simulink model "ACtoDC_WPT_DC_two_phase"  (R2018a)
settings: Solver=FixedStepAuto  StartTime=0.0  StopTime=stopTime  FixedStep=sampleTime  RelTol=1e-3
InitFcn:
  | fs=150e3; %Hz
  | wo=2*pi*fs;
  | stopTime=0.1;
  | sampleTime=1e-8;
  | Lp=81e-6;
  | Lp=32e-6;
  | Ls=66e-6;
  | Cs=1/ (Ls*4*pi*pi*150e3*150e3);
  | Cp=1/ (Lp*4*pi*pi*150e3*150e3);
  | RLOAD=20
  | RLOAD=16.2
  | k=0.2;
  | M=sqrt(Lp*Ls)*k;
  | Cout=1e-6; %F
  | fs=150e3*sqrt(1+k^2); %Hz
  | Rp=0.2
libraries: powerlib x94, simulink x6, dspstat3 x1
settings Model: Creator=enes_  LastModifiedBy=enes_

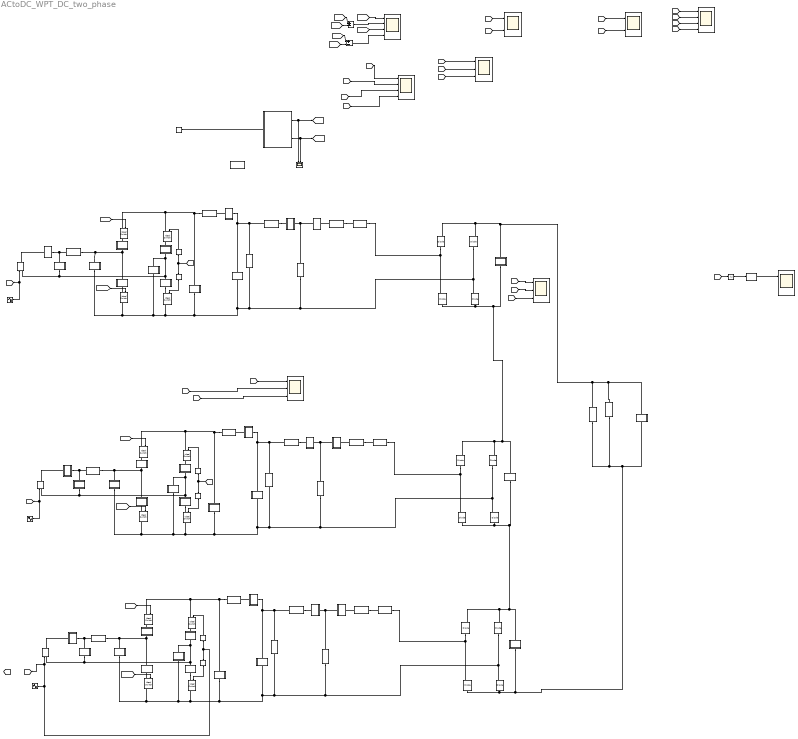
== system ACtoDC_WPT_DC_two_phase ==
  Abs : Abs
  C_TX : Subsystem
  C_TX1 : Subsystem
  C_TX10 : Subsystem
  C_TX11 : Subsystem
  C_TX12 : Subsystem
  C_TX13 : Subsystem
  C_TX14 : Subsystem
  C_TX15 : Subsystem
  C_TX16 : Subsystem
  C_TX17 : Subsystem
  C_TX18 : Subsystem
  C_TX19 : Subsystem
  C_TX2 : Subsystem
  C_TX20 : Subsystem
  C_TX21 : Subsystem
  C_TX22 : Subsystem
  C_TX23 : Subsystem
  C_TX3 : Subsystem
  C_TX4 : Subsystem
  C_TX5 : Subsystem
  C_TX6 : Subsystem
  C_TX7 : Subsystem
  C_TX8 : Subsystem
  C_TX9 : Subsystem
  Compare To Zero : simulink/Logic and Bit Operations/Compare To Zero  relop=<=  OutDataTypeStr=boolean
  Compare To Zero1 : simulink/Logic and Bit Operations/Compare To Zero  relop=>=  OutDataTypeStr=boolean
  Compare To Zero2 : simulink/Logic and Bit Operations/Compare To Zero  relop=<=  OutDataTypeStr=boolean
  Compare To Zero3 : simulink/Logic and Bit Operations/Compare To Zero  relop=>=  OutDataTypeStr=boolean
  Compare To Zero4 : simulink/Logic and Bit Operations/Compare To Zero  relop=<=  OutDataTypeStr=boolean
  Compare To Zero5 : simulink/Logic and Bit Operations/Compare To Zero  relop=>=  OutDataTypeStr=boolean
  Constant2 : Constant  Value=fs
  Controlled Voltage Source : powerlib/Electrical Sources/Controlled Voltage Source  Initialize=on  Source_Type=AC  Amplitude=0  Phase=0  Frequency=0  Measurements=None
  Controlled Voltage Source1 : powerlib/Electrical Sources/Controlled Voltage Source  Initialize=on  Source_Type=AC  Amplitude=0  Phase=0  Frequency=0  Measurements=None
  Controlled Voltage Source2 : powerlib/Electrical Sources/Controlled Voltage Source  Initialize=on  Source_Type=AC  Amplitude=0  Phase=0  Frequency=0  Measurements=None
  Diode{,1..11} (12 alike) : powerlib/Power Electronics/Diode  Ron=0.001  Lon=0  Vf=0.8  IC=0  UseSnubber=0  Rs=500  Cs=250e-9  Measurements=on
  Ideal Switch{,1..11} (12 alike) : powerlib/Power Electronics/Ideal Switch  Ron=0.01  Lon=0  IC=0  Rs=1e5  Cs=inf  Measurements=on
  Mean : dspstat3/Mean  run=on  InputProcessing=Columns as channels (frame based)  reset_popup=None  directionMode=Each column  dimension=1  roiEnable=off  roiType=Rectangles  roiPortion=Entire ROI  roiOutput=Individual statistics for each ROI  roiFlag=off  roundingMode=Floor  overflowMode=off  outputDataTypeStr=Inherit: Same as accumulator  outputMin=[]  outputMax=[]  outputLastDataTypeStr=Inherit: Same as accumulator
  Minus : Sum  Inputs=+-
  Minus1 : Sum  Inputs=+-
  Scope1 : Scope  NumInputPorts=2
  Series RLC Branch1 : powerlib/Elements/Series RLC Branch  LConnTagsString=__new0  RConnTagsString=__new0  BranchType=R  Resistance=RLOAD/2  Inductance=Lp  SetiL0=off  InitialCurrent=0  Capacitance=Cp  Setx0=off  InitialVoltage=0  Measurements=None
  Series RLC Branch10 : powerlib/Elements/Series RLC Branch  LConnTagsString=__new0  RConnTagsString=__new0  BranchType=R  Resistance=0.01  Inductance=Lp  SetiL0=off  InitialCurrent=0  Capacitance=0.01  Setx0=off  InitialVoltage=0  Measurements=None
  Series RLC Branch11 : powerlib/Elements/Series RLC Branch  LConnTagsString=__new0  RConnTagsString=__new0  BranchType=L  Resistance=Rp  Inductance=Lp-M  SetiL0=off  InitialCurrent=0  Capacitance=Cp  Setx0=off  InitialVoltage=0  Measurements=None
  Series RLC Branch12 : powerlib/Elements/Series RLC Branch  LConnTagsString=__new0  RConnTagsString=__new0  BranchType=L  Resistance=Rp  Inductance=M  SetiL0=off  InitialCurrent=0  Capacitance=Cp  Setx0=off  InitialVoltage=0  Measurements=None
  Series RLC Branch13 : powerlib/Elements/Series RLC Branch  LConnTagsString=__new0  RConnTagsString=__new0  BranchType=R  Resistance=0.01  Inductance=Lp  SetiL0=off  InitialCurrent=0  Capacitance=0.01  Setx0=off  InitialVoltage=0  Measurements=None
  Series RLC Branch14 : powerlib/Elements/Series RLC Branch  LConnTagsString=__new0  RConnTagsString=__new0  BranchType=C  Resistance=Rp  Inductance=Lp  SetiL0=off  InitialCurrent=0  Capacitance=Cp  Setx0=off  InitialVoltage=0  Measurements=None
  Series RLC Branch15 : powerlib/Elements/Series RLC Branch  LConnTagsString=__new0  RConnTagsString=__new0  BranchType=L  Resistance=Rp  Inductance=Ls-M  SetiL0=off  InitialCurrent=0  Capacitance=Cp  Setx0=off  InitialVoltage=0  Measurements=None
  Series RLC Branch16 : powerlib/Elements/Series RLC Branch  LConnTagsString=__new0  RConnTagsString=__new0  BranchType=C  Resistance=Rp  Inductance=Lp  SetiL0=off  InitialCurrent=0  Capacitance=Cs  Setx0=off  InitialVoltage=0  Measurements=None
  Series RLC Branch17 : powerlib/Elements/Series RLC Branch  LConnTagsString=__new0  RConnTagsString=__new0  BranchType=RL  Resistance=Rp  Inductance=1500e-6  SetiL0=off  InitialCurrent=0  Capacitance=Cp  Setx0=off  InitialVoltage=0  Measurements=None
  Series RLC Branch18 : powerlib/Elements/Series RLC Branch  LConnTagsString=__new0  RConnTagsString=__new0  BranchType=R  Resistance=0.01  Inductance=Lp  SetiL0=off  InitialCurrent=0  Capacitance=0.01  Setx0=off  InitialVoltage=0  Measurements=None
  Series RLC Branch19 : powerlib/Elements/Series RLC Branch  LConnTagsString=__new0  RConnTagsString=__new0  BranchType=L  Resistance=Rp  Inductance=Lp-M  SetiL0=off  InitialCurrent=0  Capacitance=Cp  Setx0=off  InitialVoltage=0  Measurements=None
  Series RLC Branch2 : powerlib/Elements/Series RLC Branch  LConnTagsString=__new0  RConnTagsString=__new0  BranchType=L  Resistance=Rp  Inductance=Lp-M  SetiL0=off  InitialCurrent=0  Capacitance=Cp  Setx0=off  InitialVoltage=0  Measurements=None
  Series RLC Branch20 : powerlib/Elements/Series RLC Branch  LConnTagsString=__new0  RConnTagsString=__new0  BranchType=L  Resistance=Rp  Inductance=M  SetiL0=off  InitialCurrent=0  Capacitance=Cp  Setx0=off  InitialVoltage=0  Measurements=None
  Series RLC Branch21 : powerlib/Elements/Series RLC Branch  LConnTagsString=__new0  RConnTagsString=__new0  BranchType=C  Resistance=Rp  Inductance=Lp  SetiL0=off  InitialCurrent=0  Capacitance=Cp  Setx0=off  InitialVoltage=0  Measurements=None
  Series RLC Branch22 : powerlib/Elements/Series RLC Branch  LConnTagsString=__new0  RConnTagsString=__new0  BranchType=L  Resistance=Rp  Inductance=Ls-M  SetiL0=off  InitialCurrent=0  Capacitance=Cp  Setx0=off  InitialVoltage=0  Measurements=None
  Series RLC Branch23 : powerlib/Elements/Series RLC Branch  LConnTagsString=__new0  RConnTagsString=__new0  BranchType=C  Resistance=Rp  Inductance=Lp  SetiL0=off  InitialCurrent=0  Capacitance=Cs  Setx0=off  InitialVoltage=0  Measurements=None
  Series RLC Branch24 : powerlib/Elements/Series RLC Branch  LConnTagsString=__new0  RConnTagsString=__new0  BranchType=RL  Resistance=Rp  Inductance=1500e-6  SetiL0=off  InitialCurrent=0  Capacitance=Cp  Setx0=off  InitialVoltage=0  Measurements=None
  Series RLC Branch3 : powerlib/Elements/Series RLC Branch  LConnTagsString=__new0  RConnTagsString=__new0  BranchType=L  Resistance=Rp  Inductance=M  SetiL0=off  InitialCurrent=0  Capacitance=Cp  Setx0=off  InitialVoltage=0  Measurements=None
  Series RLC Branch4 : powerlib/Elements/Series RLC Branch  LConnTagsString=__new0  RConnTagsString=__new0  BranchType=C  Resistance=Rp  Inductance=Lp  SetiL0=off  InitialCurrent=0  Capacitance=Cp  Setx0=off  InitialVoltage=0  Measurements=None
  Series RLC Branch5 : powerlib/Elements/Series RLC Branch  LConnTagsString=__new0  RConnTagsString=__new0  BranchType=L  Resistance=Rp  Inductance=Ls-M  SetiL0=off  InitialCurrent=0  Capacitance=Cp  Setx0=off  InitialVoltage=0  Measurements=None
  Series RLC Branch6 : powerlib/Elements/Series RLC Branch  LConnTagsString=__new0  RConnTagsString=__new0  BranchType=C  Resistance=Rp  Inductance=Lp  SetiL0=off  InitialCurrent=0  Capacitance=Cs  Setx0=off  InitialVoltage=0  Measurements=None
  Series RLC Branch7 : powerlib/Elements/Series RLC Branch  LConnTagsString=__new0  RConnTagsString=__new0  BranchType=RL  Resistance=Rp  Inductance=1500e-6  SetiL0=off  InitialCurrent=0  Capacitance=Cp  Setx0=off  InitialVoltage=0  Measurements=None
  Series RLC Branch8 : powerlib/Elements/Series RLC Branch  LConnTagsString=__new0  RConnTagsString=__new0  BranchType=C  Resistance=RLOAD  Inductance=Lp  SetiL0=off  InitialCurrent=0  Capacitance=10e-6  Setx0=off  InitialVoltage=0  Measurements=None
  Sine Wave : Sin  Amplitude=50  Frequency=2*pi*50  SampleTime=0
  Sine Wave1 : Sin  Amplitude=50  Frequency=2*pi*50  Phase=2*pi/3  SampleTime=0
  Sine Wave2 : Sin  Amplitude=50  Frequency=2*pi*50  Phase=-2*pi/3  SampleTime=0
  Subsystem1 : Subsystem
  V-I Measurement1 : Scope  NumInputPorts=3
  V-I Measurement2 : Scope  NumInputPorts=2
  V-I Measurement3 : Scope  NumInputPorts=3
  V-I Measurement4 : Scope  NumInputPorts=3
  V-I Measurement5 : Scope  NumInputPorts=2
  V-I Measurement6 : Scope  NumInputPorts=4
  V-I Measurement7 : Scope  NumInputPorts=4
  V-I Measurement8 : Scope  NumInputPorts=2
  V-I Measurement9 : Scope  NumInputPorts=4
  V_HB : Subsystem
  V_HB1 : Subsystem
  V_HB10 : Subsystem
  V_HB11 : Subsystem
  V_HB12 : Subsystem
  V_HB13 : Subsystem
  V_HB14 : Subsystem
  V_HB15 : Subsystem
  V_HB16 : Subsystem
  V_HB17 : Subsystem
  V_HB18 : Subsystem
  V_HB2 : Subsystem
  V_HB3 : Subsystem
  V_HB4 : Subsystem
  V_HB5 : Subsystem
  V_HB6 : Subsystem
  V_HB7 : Subsystem
  V_HB8 : Subsystem
  V_HB9 : Subsystem
  powergui : powerlib/powergui  Priority=1  SimulationMode=Discrete  SampleTime=sampleTime  frequency=60  Iterations=50  frequencyindice=0  Pbase=100e6  ErrMax=1e-4  UnitsV=kV  UnitsW=MW  buscounter=0  FunctionMessages=off  echomessages=off  EnableUseOfTLC=off  CurrentSourceSwitches=off  DisableSnubberDevices=off  DisableRonSwitches=off  DisableVfSwitches=off  DisplayEquations=off  SolverType=Tustin/Backward Euler (TBE)  Interpol=off  ExternalGateDelay=off  methode=off  Ts=100  x0status=blocks  SPID=off  SwTol=0  HookPort=off  RestoreLinks=warning  ResistiveCurrentMeasurement=off  Frange=[0:2:500]  Ylog=off  Xlog=on  ShowGrid=off  save=off  variable=ZData  structure=ScopeData10  ZoomFFT=off  StartTime=0.0  cycles=2  DisplayStyle=2  fundamental=50  FreqAxis=off  MaxFrequency=100e3  frequencyindicesteady=1  RmsSteady=1  display=off
  tag scope: PWMA_TOP=global
  wires:
  [V_in] -> V-I Measurement5/2  "Vin"
  Subsystem1/2(PWMA_BOT) -> Scope1/2, [PWMA_BOT]  "TA-"
  Subsystem1/1(PWMA_TOP) -> [PWMA_TOP], Scope1/1  "TA+"
  [V_aminus] -> V-I Measurement6/1  "Va-"
  [V_aposmin] -> Minus/1
  [V_aminus] -> Minus/2
  Minus/1 -> V-I Measurement6/2  "Va+"
  [V_bminus] -> V-I Measurement6/3  "Vb-"
  [V_aposmin] -> Minus1/1
  [V_bminus] -> Minus1/2
  Minus1/1 -> V-I Measurement6/4  "Vb+"
  [I_apos] -> V-I Measurement7/1  "Ia+"
  [I_bpos] -> V-I Measurement7/2  "Ib+"
  [I_in] -> V-I Measurement5/1  "Iin"
  [V_HB] -> V-I Measurement8/1  "VHB"
  [I_HB] -> V-I Measurement8/2  "IHB"
  [V_HB] -> V-I Measurement9/1  "Vtx"
  [I_Tx] -> V-I Measurement9/2  "Itx"
  [I_Rx] -> V-I Measurement9/3  "Irx"
  [Vout] -> V-I Measurement9/4  "Vrx"
  [V_in] -> V-I Measurement1/1  "Vin"
  [Vout] -> V-I Measurement1/3  "Vout"
  [I_in] -> V-I Measurement1/2  "Iin"
  [I_bmin] -> V-I Measurement7/3  "Ib-"
  [I_amin] -> V-I Measurement7/4  "Ia-"
  Constant2/1 -> Subsystem1/1(Frequency)
  Sine Wave/1 -> [Vin], Controlled Voltage Source/1
  Compare To Zero1/1 -> Ideal Switch2/1
  Mean/1 -> V-I Measurement2/1
  [Vin] -> Compare To Zero1/1, Compare To Zero/1
  [Vout] -> Abs/1
  Abs/1 -> Mean/1
  [PWMA_BOT] -> Ideal Switch/1
  [PWMA_TOP] -> Ideal Switch1/1
  Compare To Zero/1 -> Ideal Switch3/1
  [Vin2] -> Compare To Zero3/1, Compare To Zero2/1
  Compare To Zero2/1 -> Ideal Switch7/1
  [PWMA_BOT] -> Ideal Switch4/1
  [PWMA_TOP] -> Ideal Switch5/1
  Sine Wave1/1 -> [Vin2], Controlled Voltage Source1/1
  Compare To Zero3/1 -> Ideal Switch6/1
  [Vout1] -> V-I Measurement3/1
  [Vout2] -> V-I Measurement3/2
  [Vout] -> V-I Measurement3/3
  Compare To Zero5/1 -> Ideal Switch10/1
  [PWMA_TOP] -> Ideal Switch9/1
  Sine Wave2/1 -> [Vin3], Controlled Voltage Source2/1, Compare To Zero5/1, Compare To Zero4/1
  [PWMA_BOT] -> Ideal Switch8/1
  Compare To Zero4/1 -> Ideal Switch11/1
  [I_in] -> V-I Measurement4/1  "Iin"
  [I_in2] -> V-I Measurement4/2
  [I_in3] -> V-I Measurement4/3
  connections:
  Ideal Switch/RConn1 -- Diode3/RConn1 -- Diode2/LConn1 -- Series RLC Branch3/RConn1 -- Series RLC Branch4/RConn1 -- V_HB/LConn1 -- V_HB2/LConn1 -- Ideal Switch2/RConn1 -- V_HB3/LConn1 -- V_HB7/LConn1
  Series RLC Branch4/LConn1 -- V_HB/RConn1 -- C_TX4/RConn1 -- Series RLC Branch2/LConn1
  V_HB6/RConn1 -- C_TX6/RConn1 -- Series RLC Branch7/LConn1
  Series RLC Branch13/RConn1 -- Ideal Switch1/LConn1 -- Ideal Switch3/LConn1 -- V_HB2/RConn1
  C_TX/RConn1 -- Series RLC Branch3/LConn1 -- C_TX1/LConn1
  V_HB7/RConn1 -- Series RLC Branch7/RConn1 -- C_TX5/LConn1 -- C_TX2/LConn1
  Diode/LConn1 -- Series RLC Branch6/LConn1 -- Diode1/RConn1
  Series RLC Branch5/LConn1 -- C_TX1/RConn1
  Series RLC Branch2/RConn1 -- C_TX/LConn1
  C_TX2/RConn1 -- Ideal Switch1/RConn1
  C_TX4/LConn1 -- Series RLC Branch13/LConn1
  C_TX3/RConn1 -- Ideal Switch3/RConn1
  C_TX7/RConn1 -- Ideal Switch2/LConn1
  Series RLC Branch5/RConn1 -- Series RLC Branch6/RConn1
  Ideal Switch/LConn1 -- C_TX5/RConn1
  Controlled Voltage Source/RConn1 -- C_TX6/LConn1
  Ideal Switch4/RConn1 -- V_HB11/LConn1 -- V_HB9/LConn1 -- Ideal Switch6/RConn1 -- V_HB8/LConn1 -- V_HB4/LConn1 -- Series RLC Branch14/RConn1 -- Series RLC Branch12/RConn1 -- Diode7/RConn1 -- Diode6/LConn1
  Diode4/LConn1 -- Series RLC Branch16/LConn1 -- Diode5/RConn1
  Series RLC Branch10/RConn1 -- Ideal Switch5/LConn1 -- Ideal Switch7/LConn1 -- V_HB8/RConn1
  C_TX8/RConn1 -- Series RLC Branch12/LConn1 -- C_TX9/LConn1
  V_HB11/RConn1 -- Series RLC Branch17/RConn1 -- C_TX13/LConn1 -- C_TX10/LConn1
  Diode8/RConn1 -- V_HB16/RConn1 -- V_HB5/LConn1 -- Diode5/LConn1 -- Diode7/LConn1 -- Diode10/RConn1
  Series RLC Branch14/LConn1 -- Series RLC Branch11/LConn1 -- V_HB4/RConn1 -- C_TX12/RConn1
  V_HB10/RConn1 -- C_TX14/RConn1 -- Series RLC Branch17/LConn1
  Series RLC Branch15/RConn1 -- Series RLC Branch16/RConn1
  Series RLC Branch11/RConn1 -- C_TX8/LConn1
  C_TX12/LConn1 -- Series RLC Branch10/LConn1
  Series RLC Branch15/LConn1 -- C_TX9/RConn1
  C_TX11/RConn1 -- Ideal Switch7/RConn1
  C_TX10/RConn1 -- Ideal Switch5/RConn1
  C_TX15/RConn1 -- Ideal Switch6/LConn1
  Ideal Switch4/LConn1 -- C_TX13/RConn1
  C_TX17/LConn1 -- Controlled Voltage Source2/LConn1 -- V_HB13/LConn1 -- C_TX21/LConn1 -- V_HB18/RConn1
  V_HB14/RConn1 -- Series RLC Branch24/RConn1 -- C_TX19/LConn1 -- C_TX16/LConn1
  C_TX22/RConn1 -- Series RLC Branch20/LConn1 -- C_TX23/LConn1
  V_HB13/RConn1 -- C_TX20/RConn1 -- Series RLC Branch24/LConn1
  Ideal Switch8/RConn1 -- V_HB14/LConn1 -- V_HB18/LConn1 -- Ideal Switch10/RConn1 -- V_HB17/LConn1 -- V_HB15/LConn1 -- Series RLC Branch21/RConn1 -- Series RLC Branch20/RConn1 -- Diode11/RConn1 -- Diode10/LConn1
  Series RLC Branch18/RConn1 -- V_HB17/RConn1 -- Ideal Switch9/LConn1 -- Ideal Switch11/LConn1
  C_TX18/RConn1 -- V_HB15/RConn1 -- Series RLC Branch19/LConn1 -- Series RLC Branch21/LConn1
  Diode8/LConn1 -- Series RLC Branch23/LConn1 -- Diode9/RConn1
  C_TX17/RConn1 -- Ideal Switch11/RConn1
  Ideal Switch8/LConn1 -- C_TX19/RConn1
  Series RLC Branch22/RConn1 -- Series RLC Branch23/RConn1
  Series RLC Branch19/RConn1 -- C_TX22/LConn1
  C_TX21/RConn1 -- Ideal Switch10/LConn1
  C_TX18/LConn1 -- Series RLC Branch18/LConn1
  Controlled Voltage Source2/RConn1 -- C_TX20/LConn1
  Series RLC Branch22/LConn1 -- C_TX23/RConn1
  C_TX16/RConn1 -- Ideal Switch9/RConn1
  Diode/RConn1 -- Series RLC Branch8/LConn1 -- Series RLC Branch1/LConn1 -- V_HB12/RConn1 -- V_HB1/RConn1 -- Diode2/RConn1
  Series RLC Branch1/RConn1 -- Series RLC Branch8/RConn1 -- Diode9/LConn1 -- Diode11/LConn1 -- V_HB16/LConn1 -- V_HB12/LConn1
  Controlled Voltage Source1/RConn1 -- C_TX14/LConn1
  V_HB6/LConn1 -- Controlled Voltage Source/LConn1 -- C_TX7/LConn1 -- V_HB3/RConn1 -- C_TX3/LConn1
  V_HB10/LConn1 -- Controlled Voltage Source1/LConn1 -- C_TX15/LConn1 -- V_HB9/RConn1 -- C_TX11/LConn1
  V_HB1/LConn1 -- V_HB5/RConn1 -- Diode6/RConn1 -- Diode4/RConn1 -- Diode1/LConn1 -- Diode3/LConn1

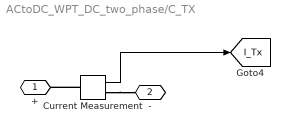
== system ACtoDC_WPT_DC_two_phase/C_TX ==
  Current Measurement : powerlib/Measurements/Current Measurement  PhasorSimulation=off  OutputType=Complex  PSBequivalent=0
  + : PMIOPort  Side=Left
  - : PMIOPort  Port=2  Side=Right
  tag scope: I_Tx=global
  wires:
  Current Measurement/1 -> [I_Tx]
  connections:
  Current Measurement/RConn1 -- -/RConn1
  Current Measurement/LConn1 -- +/RConn1

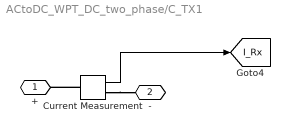
== system ACtoDC_WPT_DC_two_phase/C_TX1 ==
  Current Measurement : powerlib/Measurements/Current Measurement  PhasorSimulation=off  OutputType=Complex  PSBequivalent=0
  + : PMIOPort  Side=Left
  - : PMIOPort  Port=2  Side=Right
  tag scope: I_Rx=global
  wires:
  Current Measurement/1 -> [I_Rx]
  connections:
  Current Measurement/RConn1 -- -/RConn1
  Current Measurement/LConn1 -- +/RConn1

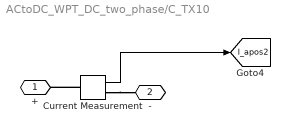
== system ACtoDC_WPT_DC_two_phase/C_TX10 ==
  Current Measurement : powerlib/Measurements/Current Measurement  PhasorSimulation=off  OutputType=Complex  PSBequivalent=0
  + : PMIOPort  Side=Left
  - : PMIOPort  Port=2  Side=Right
  tag scope: I_apos2=global
  wires:
  Current Measurement/1 -> [I_apos2]
  connections:
  Current Measurement/RConn1 -- -/RConn1
  Current Measurement/LConn1 -- +/RConn1

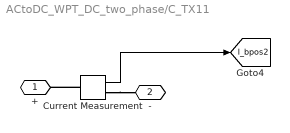
== system ACtoDC_WPT_DC_two_phase/C_TX11 ==
  Current Measurement : powerlib/Measurements/Current Measurement  PhasorSimulation=off  OutputType=Complex  PSBequivalent=0
  + : PMIOPort  Side=Left
  - : PMIOPort  Port=2  Side=Right
  tag scope: I_bpos2=global
  wires:
  Current Measurement/1 -> [I_bpos2]
  connections:
  Current Measurement/RConn1 -- -/RConn1
  Current Measurement/LConn1 -- +/RConn1

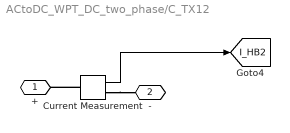
== system ACtoDC_WPT_DC_two_phase/C_TX12 ==
  Current Measurement : powerlib/Measurements/Current Measurement  PhasorSimulation=off  OutputType=Complex  PSBequivalent=0
  + : PMIOPort  Side=Left
  - : PMIOPort  Port=2  Side=Right
  tag scope: I_HB2=global
  wires:
  Current Measurement/1 -> [I_HB2]
  connections:
  Current Measurement/RConn1 -- -/RConn1
  Current Measurement/LConn1 -- +/RConn1

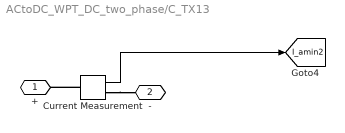
== system ACtoDC_WPT_DC_two_phase/C_TX13 ==
  Current Measurement : powerlib/Measurements/Current Measurement  PhasorSimulation=off  OutputType=Complex  PSBequivalent=0
  + : PMIOPort  Side=Left
  - : PMIOPort  Port=2  Side=Right
  tag scope: I_amin2=global
  wires:
  Current Measurement/1 -> [I_amin2]
  connections:
  Current Measurement/RConn1 -- -/RConn1
  Current Measurement/LConn1 -- +/RConn1

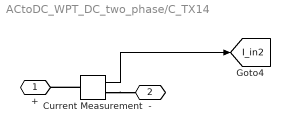
== system ACtoDC_WPT_DC_two_phase/C_TX14 ==
  Current Measurement : powerlib/Measurements/Current Measurement  PhasorSimulation=off  OutputType=Complex  PSBequivalent=0
  + : PMIOPort  Side=Left
  - : PMIOPort  Port=2  Side=Right
  tag scope: I_in2=global
  wires:
  Current Measurement/1 -> [I_in2]
  connections:
  Current Measurement/RConn1 -- -/RConn1
  Current Measurement/LConn1 -- +/RConn1

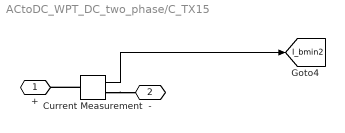
== system ACtoDC_WPT_DC_two_phase/C_TX15 ==
  Current Measurement : powerlib/Measurements/Current Measurement  PhasorSimulation=off  OutputType=Complex  PSBequivalent=0
  + : PMIOPort  Side=Left
  - : PMIOPort  Port=2  Side=Right
  tag scope: I_bmin2=global
  wires:
  Current Measurement/1 -> [I_bmin2]
  connections:
  Current Measurement/RConn1 -- -/RConn1
  Current Measurement/LConn1 -- +/RConn1

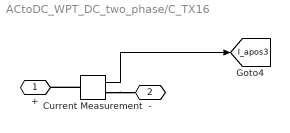
== system ACtoDC_WPT_DC_two_phase/C_TX16 ==
  Current Measurement : powerlib/Measurements/Current Measurement  PhasorSimulation=off  OutputType=Complex  PSBequivalent=0
  + : PMIOPort  Side=Left
  - : PMIOPort  Port=2  Side=Right
  tag scope: I_apos3=global
  wires:
  Current Measurement/1 -> [I_apos3]
  connections:
  Current Measurement/RConn1 -- -/RConn1
  Current Measurement/LConn1 -- +/RConn1

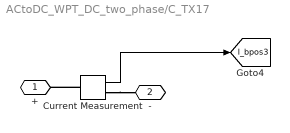
== system ACtoDC_WPT_DC_two_phase/C_TX17 ==
  Current Measurement : powerlib/Measurements/Current Measurement  PhasorSimulation=off  OutputType=Complex  PSBequivalent=0
  + : PMIOPort  Side=Left
  - : PMIOPort  Port=2  Side=Right
  tag scope: I_bpos3=global
  wires:
  Current Measurement/1 -> [I_bpos3]
  connections:
  Current Measurement/RConn1 -- -/RConn1
  Current Measurement/LConn1 -- +/RConn1

== system ACtoDC_WPT_DC_two_phase/C_TX18 ==
  Current Measurement : powerlib/Measurements/Current Measurement  PhasorSimulation=off  OutputType=Complex  PSBequivalent=0
  + : PMIOPort  Side=Left
  - : PMIOPort  Port=2  Side=Right
  tag scope: I_HB3=global
  wires:
  Current Measurement/1 -> [I_HB3]
  connections:
  Current Measurement/RConn1 -- -/RConn1
  Current Measurement/LConn1 -- +/RConn1

== system ACtoDC_WPT_DC_two_phase/C_TX19 ==
  Current Measurement : powerlib/Measurements/Current Measurement  PhasorSimulation=off  OutputType=Complex  PSBequivalent=0
  + : PMIOPort  Side=Left
  - : PMIOPort  Port=2  Side=Right
  tag scope: I_amin3=global
  wires:
  Current Measurement/1 -> [I_amin3]
  connections:
  Current Measurement/RConn1 -- -/RConn1
  Current Measurement/LConn1 -- +/RConn1

== system ACtoDC_WPT_DC_two_phase/C_TX2 ==
  Current Measurement : powerlib/Measurements/Current Measurement  PhasorSimulation=off  OutputType=Complex  PSBequivalent=0
  + : PMIOPort  Side=Left
  - : PMIOPort  Port=2  Side=Right
  tag scope: I_apos=global
  wires:
  Current Measurement/1 -> [I_apos]
  connections:
  Current Measurement/RConn1 -- -/RConn1
  Current Measurement/LConn1 -- +/RConn1

== system ACtoDC_WPT_DC_two_phase/C_TX20 ==
  Current Measurement : powerlib/Measurements/Current Measurement  PhasorSimulation=off  OutputType=Complex  PSBequivalent=0
  + : PMIOPort  Side=Left
  - : PMIOPort  Port=2  Side=Right
  tag scope: I_in3=global
  wires:
  Current Measurement/1 -> [I_in3]
  connections:
  Current Measurement/RConn1 -- -/RConn1
  Current Measurement/LConn1 -- +/RConn1

== system ACtoDC_WPT_DC_two_phase/C_TX21 ==
  Current Measurement : powerlib/Measurements/Current Measurement  PhasorSimulation=off  OutputType=Complex  PSBequivalent=0
  + : PMIOPort  Side=Left
  - : PMIOPort  Port=2  Side=Right
  tag scope: I_bmin3=global
  wires:
  Current Measurement/1 -> [I_bmin3]
  connections:
  Current Measurement/RConn1 -- -/RConn1
  Current Measurement/LConn1 -- +/RConn1

== system ACtoDC_WPT_DC_two_phase/C_TX22 ==
  Current Measurement : powerlib/Measurements/Current Measurement  PhasorSimulation=off  OutputType=Complex  PSBequivalent=0
  + : PMIOPort  Side=Left
  - : PMIOPort  Port=2  Side=Right
  tag scope: I_Tx3=global
  wires:
  Current Measurement/1 -> [I_Tx3]
  connections:
  Current Measurement/RConn1 -- -/RConn1
  Current Measurement/LConn1 -- +/RConn1

== system ACtoDC_WPT_DC_two_phase/C_TX23 ==
  Current Measurement : powerlib/Measurements/Current Measurement  PhasorSimulation=off  OutputType=Complex  PSBequivalent=0
  + : PMIOPort  Side=Left
  - : PMIOPort  Port=2  Side=Right
  tag scope: I_Rx3=global
  wires:
  Current Measurement/1 -> [I_Rx3]
  connections:
  Current Measurement/RConn1 -- -/RConn1
  Current Measurement/LConn1 -- +/RConn1

== system ACtoDC_WPT_DC_two_phase/C_TX3 ==
  Current Measurement : powerlib/Measurements/Current Measurement  PhasorSimulation=off  OutputType=Complex  PSBequivalent=0
  + : PMIOPort  Side=Left
  - : PMIOPort  Port=2  Side=Right
  tag scope: I_bpos=global
  wires:
  Current Measurement/1 -> [I_bpos]
  connections:
  Current Measurement/RConn1 -- -/RConn1
  Current Measurement/LConn1 -- +/RConn1

== system ACtoDC_WPT_DC_two_phase/C_TX4 ==
  Current Measurement : powerlib/Measurements/Current Measurement  PhasorSimulation=off  OutputType=Complex  PSBequivalent=0
  + : PMIOPort  Side=Left
  - : PMIOPort  Port=2  Side=Right
  tag scope: I_HB=global
  wires:
  Current Measurement/1 -> [I_HB]
  connections:
  Current Measurement/RConn1 -- -/RConn1
  Current Measurement/LConn1 -- +/RConn1

== system ACtoDC_WPT_DC_two_phase/C_TX5 ==
  Current Measurement : powerlib/Measurements/Current Measurement  PhasorSimulation=off  OutputType=Complex  PSBequivalent=0
  + : PMIOPort  Side=Left
  - : PMIOPort  Port=2  Side=Right
  tag scope: I_amin=global
  wires:
  Current Measurement/1 -> [I_amin]
  connections:
  Current Measurement/RConn1 -- -/RConn1
  Current Measurement/LConn1 -- +/RConn1

== system ACtoDC_WPT_DC_two_phase/C_TX6 ==
  Current Measurement : powerlib/Measurements/Current Measurement  PhasorSimulation=off  OutputType=Complex  PSBequivalent=0
  + : PMIOPort  Side=Left
  - : PMIOPort  Port=2  Side=Right
  tag scope: I_in=global
  wires:
  Current Measurement/1 -> [I_in]
  connections:
  Current Measurement/RConn1 -- -/RConn1
  Current Measurement/LConn1 -- +/RConn1

== system ACtoDC_WPT_DC_two_phase/C_TX7 ==
  Current Measurement : powerlib/Measurements/Current Measurement  PhasorSimulation=off  OutputType=Complex  PSBequivalent=0
  + : PMIOPort  Side=Left
  - : PMIOPort  Port=2  Side=Right
  tag scope: I_bmin=global
  wires:
  Current Measurement/1 -> [I_bmin]
  connections:
  Current Measurement/RConn1 -- -/RConn1
  Current Measurement/LConn1 -- +/RConn1

== system ACtoDC_WPT_DC_two_phase/C_TX8 ==
  Current Measurement : powerlib/Measurements/Current Measurement  PhasorSimulation=off  OutputType=Complex  PSBequivalent=0
  + : PMIOPort  Side=Left
  - : PMIOPort  Port=2  Side=Right
  tag scope: I_Tx2=global
  wires:
  Current Measurement/1 -> [I_Tx2]
  connections:
  Current Measurement/RConn1 -- -/RConn1
  Current Measurement/LConn1 -- +/RConn1

== system ACtoDC_WPT_DC_two_phase/C_TX9 ==
  Current Measurement : powerlib/Measurements/Current Measurement  PhasorSimulation=off  OutputType=Complex  PSBequivalent=0
  + : PMIOPort  Side=Left
  - : PMIOPort  Port=2  Side=Right
  tag scope: I_Rx2=global
  wires:
  Current Measurement/1 -> [I_Rx2]
  connections:
  Current Measurement/RConn1 -- -/RConn1
  Current Measurement/LConn1 -- +/RConn1

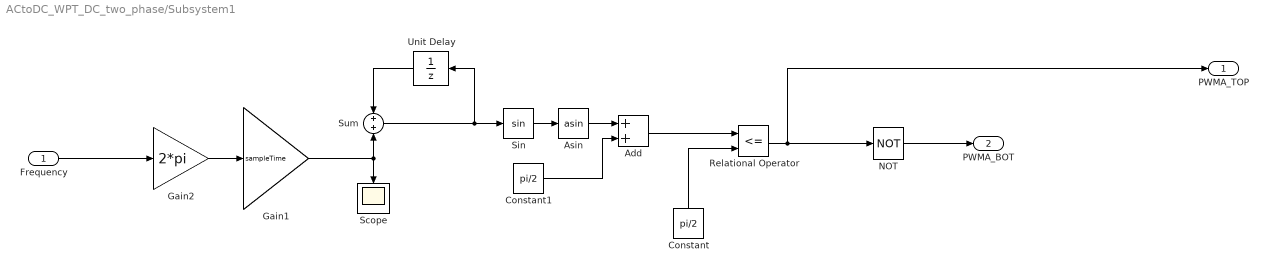
== system ACtoDC_WPT_DC_two_phase/Subsystem1 ==
  Frequency : Inport
  Add : Sum
  Asin : Trigonometry  Operator=asin
  Constant : Constant  Value=pi/2
  Constant1 : Constant  Value=pi/2
  Gain1 : Gain  Gain=sampleTime
  Gain2 : Gain  Gain=2*pi
  NOT : Logic  Operator=NOT  IconShape=distinctive  AllPortsSameDT=off  OutDataTypeStr=boolean
  Relational Operator : RelationalOperator  Operator=<=  OutDataTypeStr=boolean  RndMeth=Simplest
  Scope : Scope
  Sin : Trigonometry
  Sum : Sum
  Unit Delay : UnitDelay  SampleTime=-1
  PWMA_TOP : Outport
  PWMA_BOT : Outport  Port=2
  wires:
  Gain1/1 -> Sum/2, Scope/1
  Asin/1 -> Add/1
  Sum/1 -> Sin/1, Unit Delay/1
  Gain2/1 -> Gain1/1
  Unit Delay/1 -> Sum/1
  Relational Operator/1 -> PWMA_TOP/1, NOT/1
  Frequency/1 -> Gain2/1
  Add/1 -> Relational Operator/1
  Sin/1 -> Asin/1
  Constant1/1 -> Add/2
  Constant/1 -> Relational Operator/2
  NOT/1 -> PWMA_BOT/1

== system ACtoDC_WPT_DC_two_phase/V_HB ==
  Voltage Measurement1 : powerlib/Measurements/Voltage Measurement  PhasorSimulation=off  OutputType=Complex  PSBequivalent=0
  V+ : PMIOPort  Side=Right
  V- : PMIOPort  Port=2  Side=Left
  tag scope: V_HB=global
  wires:
  Voltage Measurement1/1 -> [V_HB]
  connections:
  Voltage Measurement1/LConn1 -- V+/RConn1
  Voltage Measurement1/LConn2 -- V-/RConn1

== system ACtoDC_WPT_DC_two_phase/V_HB1 ==
  Voltage Measurement1 : powerlib/Measurements/Voltage Measurement  PhasorSimulation=off  OutputType=Complex  PSBequivalent=0
  V+ : PMIOPort  Side=Right
  V- : PMIOPort  Port=2  Side=Left
  tag scope: Vout1=global
  wires:
  Voltage Measurement1/1 -> [Vout1]
  connections:
  Voltage Measurement1/LConn1 -- V+/RConn1
  Voltage Measurement1/LConn2 -- V-/RConn1

== system ACtoDC_WPT_DC_two_phase/V_HB10 ==
  Voltage Measurement1 : powerlib/Measurements/Voltage Measurement  PhasorSimulation=off  OutputType=Complex  PSBequivalent=0
  V+ : PMIOPort  Side=Right
  V- : PMIOPort  Port=2  Side=Left
  tag scope: V_in2=global
  wires:
  Voltage Measurement1/1 -> [V_in2]
  connections:
  Voltage Measurement1/LConn1 -- V+/RConn1
  Voltage Measurement1/LConn2 -- V-/RConn1

== system ACtoDC_WPT_DC_two_phase/V_HB11 ==
  Voltage Measurement1 : powerlib/Measurements/Voltage Measurement  PhasorSimulation=off  OutputType=Complex  PSBequivalent=0
  V+ : PMIOPort  Side=Right
  V- : PMIOPort  Port=2  Side=Left
  tag scope: V_aminus2=global
  wires:
  Voltage Measurement1/1 -> [V_aminus2]
  connections:
  Voltage Measurement1/LConn1 -- V+/RConn1
  Voltage Measurement1/LConn2 -- V-/RConn1

== system ACtoDC_WPT_DC_two_phase/V_HB12 ==
  Voltage Measurement1 : powerlib/Measurements/Voltage Measurement  PhasorSimulation=off  OutputType=Complex  PSBequivalent=0
  V+ : PMIOPort  Side=Right
  V- : PMIOPort  Port=2  Side=Left
  tag scope: Vout=global
  wires:
  Voltage Measurement1/1 -> [Vout]
  connections:
  Voltage Measurement1/LConn1 -- V+/RConn1
  Voltage Measurement1/LConn2 -- V-/RConn1

== system ACtoDC_WPT_DC_two_phase/V_HB13 ==
  Voltage Measurement1 : powerlib/Measurements/Voltage Measurement  PhasorSimulation=off  OutputType=Complex  PSBequivalent=0
  V+ : PMIOPort  Side=Right
  V- : PMIOPort  Port=2  Side=Left
  tag scope: V_in3=global
  wires:
  Voltage Measurement1/1 -> [V_in3]
  connections:
  Voltage Measurement1/LConn1 -- V+/RConn1
  Voltage Measurement1/LConn2 -- V-/RConn1

== system ACtoDC_WPT_DC_two_phase/V_HB14 ==
  Voltage Measurement1 : powerlib/Measurements/Voltage Measurement  PhasorSimulation=off  OutputType=Complex  PSBequivalent=0
  V+ : PMIOPort  Side=Right
  V- : PMIOPort  Port=2  Side=Left
  tag scope: V_aminus3=global
  wires:
  Voltage Measurement1/1 -> [V_aminus3]
  connections:
  Voltage Measurement1/LConn1 -- V+/RConn1
  Voltage Measurement1/LConn2 -- V-/RConn1

== system ACtoDC_WPT_DC_two_phase/V_HB15 ==
  Voltage Measurement1 : powerlib/Measurements/Voltage Measurement  PhasorSimulation=off  OutputType=Complex  PSBequivalent=0
  V+ : PMIOPort  Side=Right
  V- : PMIOPort  Port=2  Side=Left
  tag scope: V_HB3=global
  wires:
  Voltage Measurement1/1 -> [V_HB3]
  connections:
  Voltage Measurement1/LConn1 -- V+/RConn1
  Voltage Measurement1/LConn2 -- V-/RConn1

== system ACtoDC_WPT_DC_two_phase/V_HB16 ==
  Voltage Measurement1 : powerlib/Measurements/Voltage Measurement  PhasorSimulation=off  OutputType=Complex  PSBequivalent=0
  V+ : PMIOPort  Side=Right
  V- : PMIOPort  Port=2  Side=Left
  tag scope: Vout3=global
  wires:
  Voltage Measurement1/1 -> [Vout3]
  connections:
  Voltage Measurement1/LConn1 -- V+/RConn1
  Voltage Measurement1/LConn2 -- V-/RConn1

== system ACtoDC_WPT_DC_two_phase/V_HB17 ==
  Voltage Measurement1 : powerlib/Measurements/Voltage Measurement  PhasorSimulation=off  OutputType=Complex  PSBequivalent=0
  V+ : PMIOPort  Side=Right
  V- : PMIOPort  Port=2  Side=Left
  tag scope: V_aposmin3=global
  wires:
  Voltage Measurement1/1 -> [V_aposmin3]
  connections:
  Voltage Measurement1/LConn1 -- V+/RConn1
  Voltage Measurement1/LConn2 -- V-/RConn1

== system ACtoDC_WPT_DC_two_phase/V_HB18 ==
  Voltage Measurement1 : powerlib/Measurements/Voltage Measurement  PhasorSimulation=off  OutputType=Complex  PSBequivalent=0
  V+ : PMIOPort  Side=Right
  V- : PMIOPort  Port=2  Side=Left
  tag scope: V_bminus3=global
  wires:
  Voltage Measurement1/1 -> [V_bminus3]
  connections:
  Voltage Measurement1/LConn1 -- V+/RConn1
  Voltage Measurement1/LConn2 -- V-/RConn1

== system ACtoDC_WPT_DC_two_phase/V_HB2 ==
  Voltage Measurement1 : powerlib/Measurements/Voltage Measurement  PhasorSimulation=off  OutputType=Complex  PSBequivalent=0
  V+ : PMIOPort  Side=Right
  V- : PMIOPort  Port=2  Side=Left
  tag scope: V_aposmin=global
  wires:
  Voltage Measurement1/1 -> [V_aposmin]
  connections:
  Voltage Measurement1/LConn1 -- V+/RConn1
  Voltage Measurement1/LConn2 -- V-/RConn1

== system ACtoDC_WPT_DC_two_phase/V_HB3 ==
  Voltage Measurement1 : powerlib/Measurements/Voltage Measurement  PhasorSimulation=off  OutputType=Complex  PSBequivalent=0
  V+ : PMIOPort  Side=Right
  V- : PMIOPort  Port=2  Side=Left
  tag scope: V_bminus=global
  wires:
  Voltage Measurement1/1 -> [V_bminus]
  connections:
  Voltage Measurement1/LConn1 -- V+/RConn1
  Voltage Measurement1/LConn2 -- V-/RConn1

== system ACtoDC_WPT_DC_two_phase/V_HB4 ==
  Voltage Measurement1 : powerlib/Measurements/Voltage Measurement  PhasorSimulation=off  OutputType=Complex  PSBequivalent=0
  V+ : PMIOPort  Side=Right
  V- : PMIOPort  Port=2  Side=Left
  tag scope: V_HB2=global
  wires:
  Voltage Measurement1/1 -> [V_HB2]
  connections:
  Voltage Measurement1/LConn1 -- V+/RConn1
  Voltage Measurement1/LConn2 -- V-/RConn1

== system ACtoDC_WPT_DC_two_phase/V_HB5 ==
  Voltage Measurement1 : powerlib/Measurements/Voltage Measurement  PhasorSimulation=off  OutputType=Complex  PSBequivalent=0
  V+ : PMIOPort  Side=Right
  V- : PMIOPort  Port=2  Side=Left
  tag scope: Vout2=global
  wires:
  Voltage Measurement1/1 -> [Vout2]
  connections:
  Voltage Measurement1/LConn1 -- V+/RConn1
  Voltage Measurement1/LConn2 -- V-/RConn1

== system ACtoDC_WPT_DC_two_phase/V_HB6 ==
  Voltage Measurement1 : powerlib/Measurements/Voltage Measurement  PhasorSimulation=off  OutputType=Complex  PSBequivalent=0
  V+ : PMIOPort  Side=Right
  V- : PMIOPort  Port=2  Side=Left
  tag scope: V_in=global
  wires:
  Voltage Measurement1/1 -> [V_in]
  connections:
  Voltage Measurement1/LConn1 -- V+/RConn1
  Voltage Measurement1/LConn2 -- V-/RConn1

== system ACtoDC_WPT_DC_two_phase/V_HB7 ==
  Voltage Measurement1 : powerlib/Measurements/Voltage Measurement  PhasorSimulation=off  OutputType=Complex  PSBequivalent=0
  V+ : PMIOPort  Side=Right
  V- : PMIOPort  Port=2  Side=Left
  tag scope: V_aminus=global
  wires:
  Voltage Measurement1/1 -> [V_aminus]
  connections:
  Voltage Measurement1/LConn1 -- V+/RConn1
  Voltage Measurement1/LConn2 -- V-/RConn1

== system ACtoDC_WPT_DC_two_phase/V_HB8 ==
  Voltage Measurement1 : powerlib/Measurements/Voltage Measurement  PhasorSimulation=off  OutputType=Complex  PSBequivalent=0
  V+ : PMIOPort  Side=Right
  V- : PMIOPort  Port=2  Side=Left
  tag scope: V_aposmin2=global
  wires:
  Voltage Measurement1/1 -> [V_aposmin2]
  connections:
  Voltage Measurement1/LConn1 -- V+/RConn1
  Voltage Measurement1/LConn2 -- V-/RConn1

== system ACtoDC_WPT_DC_two_phase/V_HB9 ==
  Voltage Measurement1 : powerlib/Measurements/Voltage Measurement  PhasorSimulation=off  OutputType=Complex  PSBequivalent=0
  V+ : PMIOPort  Side=Right
  V- : PMIOPort  Port=2  Side=Left
  tag scope: V_bminus2=global
  wires:
  Voltage Measurement1/1 -> [V_bminus2]
  connections:
  Voltage Measurement1/LConn1 -- V+/RConn1
  Voltage Measurement1/LConn2 -- V-/RConn1
